simulink model "modellabolatorium0"  (R2020b)
settings: Solver=FixedStepDiscrete  StartTime=0.0  StopTime=0.0  RelTol=1e-3
undefined symbols (not defined in the file): H, W
libraries: CPOiS_SourcesSinks x4, CPOiS_General x1
settings Model: Creator=jrybarz  LastModifiedBy=jrybarz

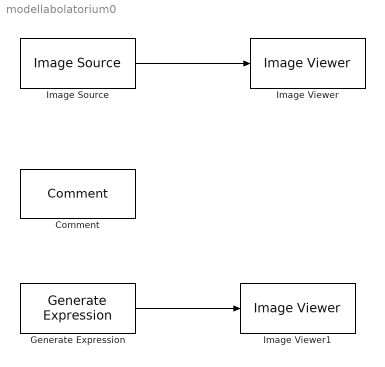
== system modellabolatorium0 ==
  Comment : CPOiS_General/Comment
      settings: SourceProductName=CPOiS - Digital image and signal processing
  Generate Expression : CPOiS_SourcesSinks/Generate Expression  Width=256  Height=256  Expression=W/2+H/2
      settings: SourceProductName=CPOiS - Digital image and signal processing
  Image Source : CPOiS_SourcesSinks/Image Source  FileSelection=rice.png
      settings: SourceProductName=CPOiS - Digital image and signal processing
  Image Viewer : CPOiS_SourcesSinks/Image Viewer
      settings: SourceProductName=CPOiS - Digital image and signal processing
  Image Viewer1 : CPOiS_SourcesSinks/Image Viewer
      settings: SourceProductName=CPOiS - Digital image and signal processing
  wires:
  Image Source/1 -> Image Viewer/1
  Generate Expression/1 -> Image Viewer1/1
